simulink model "vexv5_Clawbot_MATLAB_Driver_Safety"  (R2019a)
settings: Solver=ode3  StartTime=0.0  StopTime=inf  RelTol=1e-3  EnableMultiTasking=on
libraries: vexv5lib x9
settings Model: ExtModeTrigDuration=5  Creator=The MathWorks, Inc.  LastModifiedBy=josea
settings DataIOCC: LimitDataPoints=on  SaveFormat=Array  ReturnWorkspaceOutputs=off
settings OptimizationCC: ExpressionDepthLimit=2147483647  LifeSpan=Inf  MaxStackSize=64
settings DebuggingCC: UnderspecifiedInitializationDetection=Classic  MergeDetectMultiDrivingBlocksExec=none  InheritedTsInSrcMsg=none  FcnCallInpInsideContextMsg=warning  UnconnectedInputMsg=none  UnconnectedOutputMsg=none  AllowSymbolicDim=off  StateNameClashWarn=warning  SFUnexpectedBacktrackingDiag=warning  SFNoUnconditionalDefaultTransitionDiag=warning  SFExecutionAtInitializationDiag=none  ArithmeticOperatorsInVariantConditions=warning
settings HardwareCC: ProdBitPerPointer=32  ProdBitPerSizeT=32  ProdBitPerPtrDiffT=32  ProdLargestAtomicInteger=Long  ProdLargestAtomicFloat=Double  ProdWordSize=32  ProdHWDeviceType=ARM Compatible->ARM Cortex
settings ModelReferenceCC: PropagateSignalLabelsOutOfModel=off
settings SFSimCC: SimUseLocalCustomCode=off
settings RTWCC: SystemTargetFile=ert.tlc  HardwareBoard=VEX V5 Robot Brain  TLCOptions=-aInlineSetEventsForThisBaseRateFcn=TLC_FALSE -aSuppressMultiTaskScheduler=TLC_FALSE -aRateBasedStepFcn=0  TemplateMakefile=ert_default_tmf  RTWUseLocalCustomCode=off  Toolchain=GNU Tools for ARM Embedded Processors
settings CodeAppCC: StateflowObjectComments=on
settings ERTTargetCC: CodeReplacementLibrary=GCC ARM Cortex-M3  MultiwordLength=2048  ERTCustomFileBanners=off  SupportContinuousTime=on  SupportNonInlinedSFcns=on  RemoveResetFunc=off  ModelStepFunctionPrototypeControlCompliant=off  ConvertIfToSwitch=off  SuppressUnreachableDefaultCases=off
settings ConfigComp: CovMetricSettings=dw  CovHtmlReporting=on  CovSaveCumulativeToWorkspaceVar=on  CovSaveSingleToWorkspaceVar=on  CovExternalEMLEnable=off  CovSFcnEnable=off

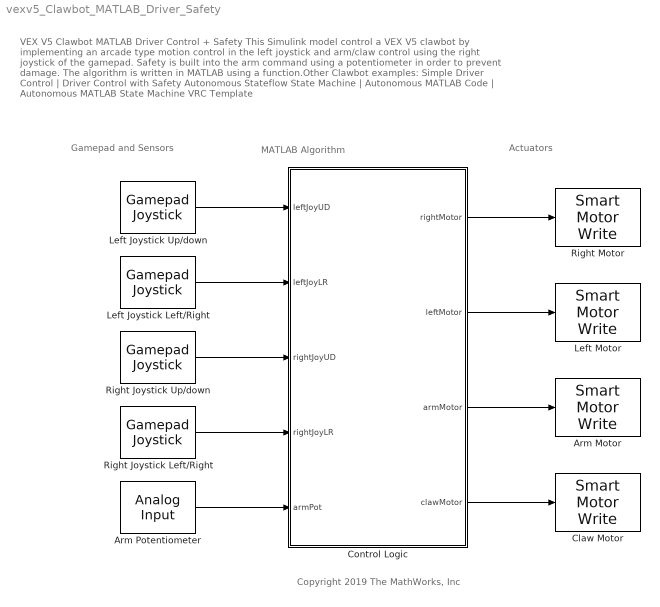
== system vexv5_Clawbot_MATLAB_Driver_Safety ==
  note: Actuators
  note: MATLAB Algorithm
  note: Gamepad and Sensors
  note: Copyright 2019 The MathWorks, Inc
  note: VEX V5 Clawbot MATLAB Driver Control + Safety
      | This Simulink model control a VEX V5 clawbot by implementing an arcade type motion control in the left joystick and arm/claw
      | control using the right joystick of the gamepad. Safety is built into the arm command using a potentiometer in order to prevent damage.
      | The algorithm is written in MATLAB using a function.Other Clawbot examples:
      | Simple Driver Control | Driver Control with Safety
      | Autonomous Stateflow State Machine | Autonomous MATLAB Code | Autonomous MATLAB State Machine
      | VRC Template
  Arm Motor : vexv5lib/Actuators/Smart Motor Write  motorPort=8  scaleFactor=18:1  MotorBrakeMode=Hold  OperationMode=Velocity Control
      settings: SourceProductName=Simulink Coder Support Package for VEX EDR V5 Robot Brain
  Arm Potentiometer : vexv5lib/Sensors/Analog Input  port=A  SampleTime=0.02
      settings: SourceProductName=Simulink Coder Support Package for VEX EDR V5 Robot Brain
  Claw Motor : vexv5lib/Actuators/Smart Motor Write  motorPort=3  scaleFactor=18:1  MotorBrakeMode=Hold  OperationMode=Velocity Control
      settings: SourceProductName=Simulink Coder Support Package for VEX EDR V5 Robot Brain
  Control Logic : MATLAB Function  TreatAsAtomicUnit=on
  Left Joystick Left/Right : vexv5lib/Gamepad/Gamepad Joystick  joystickType=Master  chan=4  SampleTime=0.02
      settings: SourceProductName=Simulink Coder Support Package for VEX EDR V5 Robot Brain
  Left Joystick Up/down : vexv5lib/Gamepad/Gamepad Joystick  joystickType=Master  chan=3  SampleTime=0.02
      settings: SourceProductName=Simulink Coder Support Package for VEX EDR V5 Robot Brain
  Left Motor : vexv5lib/Actuators/Smart Motor Write  motorPort=1  scaleFactor=18:1  MotorBrakeMode=Coast  OperationMode=Velocity Control
      settings: SourceProductName=Simulink Coder Support Package for VEX EDR V5 Robot Brain
  Right Joystick Left/Right : vexv5lib/Gamepad/Gamepad Joystick  joystickType=Master  chan=1  SampleTime=0.02
      settings: SourceProductName=Simulink Coder Support Package for VEX EDR V5 Robot Brain
  Right Joystick Up/down : vexv5lib/Gamepad/Gamepad Joystick  joystickType=Master  chan=2  SampleTime=0.02
      settings: SourceProductName=Simulink Coder Support Package for VEX EDR V5 Robot Brain
  Right Motor : vexv5lib/Actuators/Smart Motor Write  motorPort=10  scaleFactor=18:1  MotorBrakeMode=Coast  OperationMode=Velocity Control
      settings: SourceProductName=Simulink Coder Support Package for VEX EDR V5 Robot Brain
  wires:
  Right Joystick Up/down/1 -> Control Logic/3(rightJoyUD)
  Left Joystick Left/Right/1 -> Control Logic/2(leftJoyLR)
  Right Joystick Left/Right/1 -> Control Logic/4(rightJoyLR)
  Arm Potentiometer/1 -> Control Logic/5(armPot)
  Left Joystick Up/down/1 -> Control Logic/1(leftJoyUD)
  Control Logic/1(rightMotor) -> Right Motor/1
  Control Logic/2(leftMotor) -> Left Motor/1
  Control Logic/3(armMotor) -> Arm Motor/1
  Control Logic/4(clawMotor) -> Claw Motor/1

== matlab function vexv5_Clawbot_MATLAB_Driver_Safety/Control Logic ==
  data: leftJoyUD input; rightMotor output; leftJoyLR input; rightJoyUD input; rightJoyLR input; armPot input; leftMotor output; armMotor output; clawMotor output
function [rightMotor,leftMotor,armMotor,clawMotor] = robotControl(leftJoyUD, leftJoyLR, rightJoyUD, rightJoyLR, armPot)
% This MATLAB function contains the logic to map the control inputs from
% the VEX gamepad to the desired motor commands

%% Program Arcade Control for Wheels
leftMotor  = leftJoyLR + leftJoyUD;
rightMotor = leftJoyUD - leftJoyLR; 

% Saturate output to be within -127 to 127
leftMotor  = min(max(leftMotor,-127), 127);
rightMotor = min(max(rightMotor,-127), 127); 

%% Program Arm Control 
% Limit the motor command to zero if the position thresholds of the
% potentiometer are reached

if rightJoyUD > 0 && armPot < 2650 % Upper limit
    armMotor=rightJoyUD;
elseif rightJoyUD < 0 && armPot > 1400 % Lower limit
    armMotor=rightJoyUD;
else
    armMotor=0; % Motor command when limits are reached
end

% Change motor command depending on movement direction
if rightJoyUD > 0 
    armMotor = armMotor * 0.5; % More power for raising arm
else
    armMotor = armMotor * 0.3; % Less power for lowering arm
end

%% Program Claw Control

% Implement a deadzone to reduce joystick sensitivity
if rightJoyLR < 5 && rightJoyLR > -5
    clawMotor = 0;
else
    clawMotor = rightJoyLR;
end
